simulink subsystem "monocopter"  (R2023a)
settings: Solver=VariableStepAuto  StartTime=0.0  StopTime=10.0  RelTol=1e-3
settings Model: Creator=imyrsini  LastModifiedBy=imyrsini

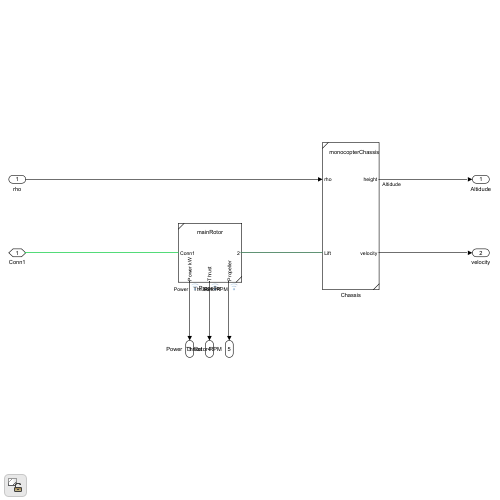
[thumbnail: Simulink's stored preview of the top-level diagram]
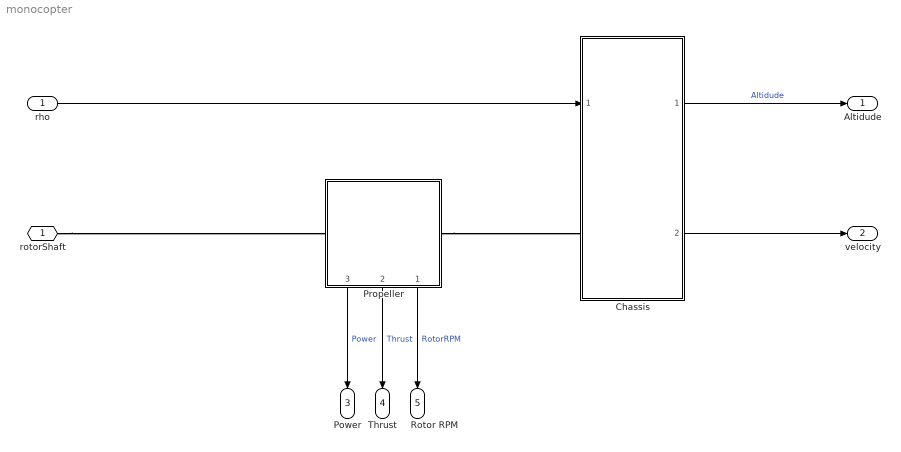
== system monocopter ==
  rho : Inport
  Chassis : Subsystem  ReferencedSubsystem=monocopterChassis
  Propeller : Subsystem  ReferencedSubsystem=mainRotor
      settings: PortSchema="{\"entries\":[{\"content\":{\"sides\":[{\"content\":{\"connectorIds\":[\"LConn1\"]},\"type\":\"ConnectorPlacement.EquallySpacedRectSide\",\"uuid\":\"dfc12c6b-9b08-4c1c-88ab-65e3cff3b522\"},{\"content\":{\"connectorIds\":[\"LConn2\"],\"side\":\"RIGHT\"},\"type\":\"ConnectorPlacement.EquallySpacedRectSide\",\"uuid\":\"ee3d6ff0-6d7f-460a-b307-c9d352a3614d\"},{\"content\":{\"side\":\"TOP\"},\"type\":\"ConnectorPlacement.EquallySpacedRectSide\",\"uuid\":\"364f8b59-b1e5-48c9-b7c4-ee70153a2521\"},{\"content\":{\"connectorIds\":[\"Out3\",\"Out2\",\"Out1\"],\"side\":\"BOTTOM\"},\"type\":\"ConnectorPlacement.EquallySpacedRectSide\",\"uuid\":\"ca79a919-3d00-4625-9426-4e8545f83d41\"}]},\"type\":\"ConnectorPlacement.EquallySpacedConnector\",\"uuid\":\"24ce1453-affd-4b81-8c92-d79bac05db4f\"}],\"packageUris\":[\"http://schema.mathworks.com/mf0/Connector/R2020b\"],\"version\":\"1.0\"}"
  rotorShaft : PMIOPort  Side=Left
  Altidude : Outport
  velocity : Outport  Port=2
  Power : Outport  Port=3
  Thrust : Outport  Port=4
  Rotor RPM : Outport  Port=5
  wires:
  Propeller/1 -> Rotor RPM/1  "RotorRPM"
  Propeller/3 -> Power/1  "Power"
  Propeller/2 -> Thrust/1  "Thrust"
  rho/1 -> Chassis/1
  Chassis/1 -> Altidude/1  "Altidude"
  Chassis/2 -> velocity/1
  connections:
  Propeller/LConn2 -- Chassis/LConn1
  rotorShaft/RConn1 -- Propeller/LConn1
